simulink model "Closed Loop Control of Separately Excited DC Motor_Block_diagram"  (R2023b)
settings: Solver=VariableStepAuto  StartTime=0.0  StopTime=2  MaxStep=1e-6  RelTol=1e-6
libraries: simulink x1, slpidlib x1
settings Model: SimulationMode=accelerator  Creator=pradnya  LastModifiedBy=Asus
settings SolverCC: AlgebraicLoopSolver=TrustRegion
settings DataIOCC: ReturnWorkspaceOutputs=off
settings DebuggingCC: UnconnectedInputMsg=warning  UnconnectedOutputMsg=warning  UnconnectedLineMsg=warning  ArithmeticOperatorsInVariantConditions=warning
settings ModelReferenceCC: EnableRefExpFcnMdlSchedulingChecks=on
settings SFSimCC: SimUseLocalCustomCode=off  CustomCodeUndefinedFunction=UseInterfaceOnly
settings RTWCC: RTWUseLocalCustomCode=off

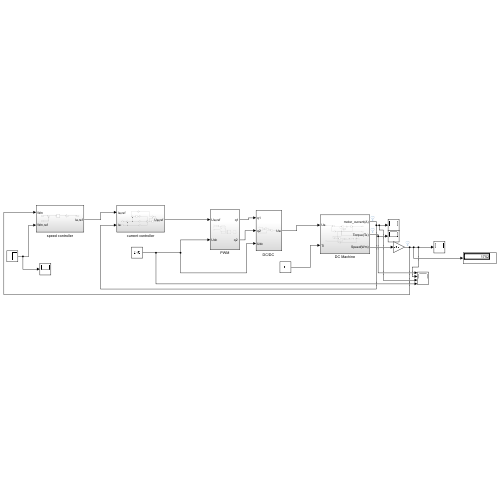
[thumbnail: Simulink's stored preview of the top-level diagram]
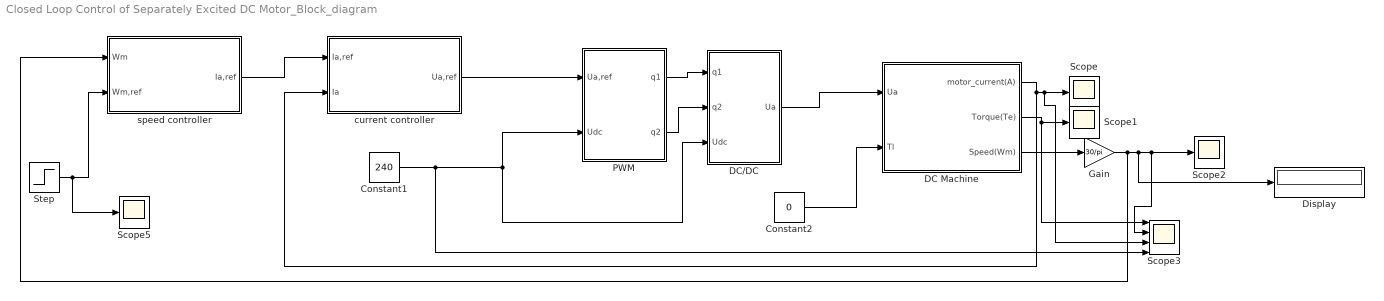
== system Closed Loop Control of Separately Excited DC Motor_Block_diagram ==
  Constant1 : Constant  Value=240
  Constant2 : Constant  Value=0
  "DC Machine " : Subsystem
  "DC/DC " : Subsystem
  Display : Display
  Gain : Gain  Gain=30/pi
  PWM : Subsystem
  Scope{,1..2,5} (4 alike) : Scope
  Scope3 : Scope  NumInputPorts=4
  Step : Step  Time=0.25  Before=875  After=1750  SampleTime=0.5
  current controller : Subsystem
  "speed controller " : Subsystem
  wires:
  "DC Machine "/3(Speed(Wm)) -> Gain/1
  "DC Machine "/2(Torque(Te)) -> Scope3/1, Scope1/1
  "DC Machine "/1(motor_current(A)) -> current controller/2(Ia), Scope3/3, Scope/1
  Gain/1 -> "speed controller "/1(Wm), Display/1, Scope3/2, Scope2/1
  PWM/1(q1) -> "DC/DC "/1(q1)
  PWM/2("q2 ") -> "DC/DC "/2(q2)
  Constant1/1 -> Scope3/4, PWM/2(Udc), "DC/DC "/3(Udc)
  Constant2/1 -> "DC Machine "/2(Tl)
  Step/1 -> Scope5/1, "speed controller "/2("Wm,ref ")
  current controller/1(Ua,ref) -> PWM/1(Ua,ref)
  "DC/DC "/1(Ua) -> "DC Machine "/1("Ua ")
  "speed controller "/1(Ia,ref) -> current controller/1("Ia,ref ")

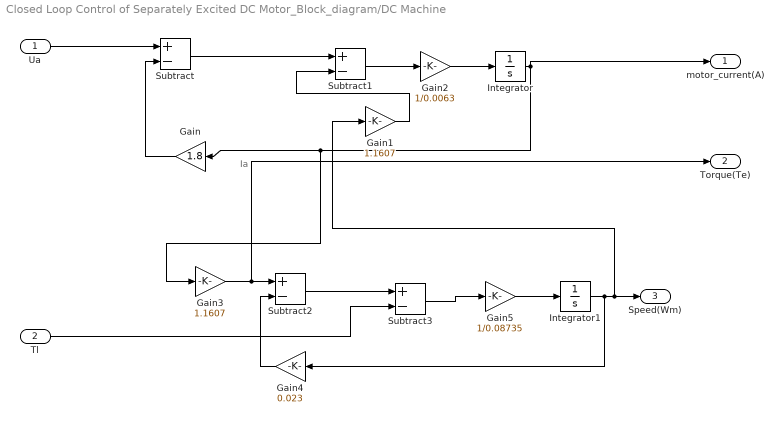
== system Closed Loop Control of Separately Excited DC Motor_Block_diagram/DC Machine  ==
  note: Ia
  "Ua " : Inport
  Tl : Inport  Port=2
  Gain : Gain  Gain=1.8
  Gain1 : Gain  Gain=1.1607
  Gain2 : Gain  Gain=1/0.0063
  Gain3 : Gain  Gain=1.1607
  Gain4 : Gain  Gain=0.023
  Gain5 : Gain  Gain=1/0.08735
  Integrator : Integrator
  Integrator1 : Integrator
  Subtract{,1..3} (4 alike) : Sum  Inputs=+-
  motor_current(A) : Outport  VectorParamsAs1DForOutWhenUnconnected=off
  Torque(Te) : Outport  Port=2  VectorParamsAs1DForOutWhenUnconnected=off
  Speed(Wm) : Outport  Port=3  VectorParamsAs1DForOutWhenUnconnected=off
  wires:
  Subtract1/1 -> Gain2/1
  Gain3/1 -> Torque(Te)/1, Subtract2/1
  Integrator/1 -> motor_current(A)/1, Gain3/1, Gain/1
  Gain2/1 -> Integrator/1
  Gain5/1 -> Integrator1/1
  Subtract/1 -> Subtract1/1
  Integrator1/1 -> Speed(Wm)/1, Gain1/1, Gain4/1
  Gain/1 -> Subtract/2
  Gain4/1 -> Subtract2/2
  Subtract2/1 -> Subtract3/1
  Subtract3/1 -> Gain5/1
  Gain1/1 -> Subtract1/2
  Tl/1 -> Subtract3/2
  "Ua "/1 -> Subtract/1

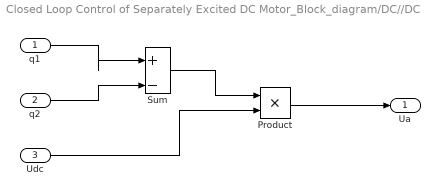
== system Closed Loop Control of Separately Excited DC Motor_Block_diagram/DC//DC  ==
  q1 : Inport
  q2 : Inport  Port=2
  Udc : Inport  Port=3
  Product : Product
  Sum : Sum  Inputs=|+-
  Ua : Outport  VectorParamsAs1DForOutWhenUnconnected=off
  wires:
  q1/1 -> Sum/1
  q2/1 -> Sum/2
  Sum/1 -> Product/1
  Udc/1 -> Product/2
  Product/1 -> Ua/1

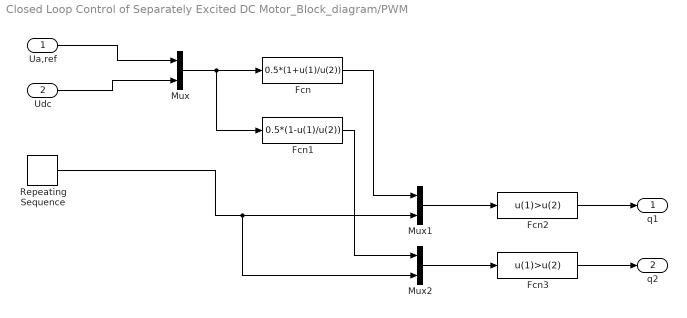
== system Closed Loop Control of Separately Excited DC Motor_Block_diagram/PWM ==
  Ua,ref : Inport
  Udc : Inport  Port=2
  Fcn : Fcn  Expr=0.5*(1+u(1)/u(2))
  Fcn1 : Fcn  Expr=0.5*(1-u(1)/u(2))
  Fcn2 : Fcn  Expr=u(1)>u(2)
  Fcn3 : Fcn  Expr=u(1)>u(2)
  Mux : Mux  Inputs=2
  Mux1 : Mux  Inputs=2
  Mux2 : Mux  Inputs=2
  Repeating Sequence : simulink/Sources/Repeating Sequence  rep_seq_t=[0 100e-6 200e-6]  rep_seq_y=[1 0 1]
  q1 : Outport  VectorParamsAs1DForOutWhenUnconnected=off
  "q2 " : Outport  Port=2  VectorParamsAs1DForOutWhenUnconnected=off
  wires:
  Ua,ref/1 -> Mux/1
  Udc/1 -> Mux/2
  Mux/1 -> Fcn1/1, Fcn/1
  Fcn/1 -> Mux1/1
  Fcn1/1 -> Mux2/1
  Repeating Sequence/1 -> Mux2/2, Mux1/2
  Mux1/1 -> Fcn2/1
  Mux2/1 -> Fcn3/1
  Fcn2/1 -> q1/1
  Fcn3/1 -> "q2 "/1

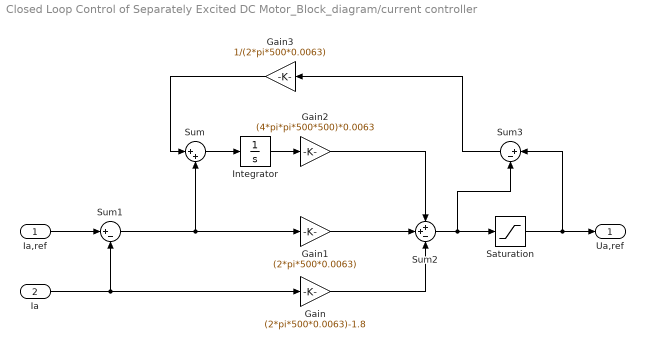
== system Closed Loop Control of Separately Excited DC Motor_Block_diagram/current controller ==
  "Ia,ref " : Inport
  Ia : Inport  Port=2
  Gain : Gain  Gain=(2*pi*500*0.0063)-1.8
  Gain1 : Gain  Gain=(2*pi*500*0.0063)
  Gain2 : Gain  Gain=(4*pi*pi*500*500)*0.0063
  Gain3 : Gain  Gain=1/(2*pi*500*0.0063)
  Integrator : Integrator
  Saturation : Saturate  UpperLimit=220  LowerLimit=-220
  Sum : Sum  Inputs=|++
  Sum1 : Sum  Inputs=|+-
  Sum2 : Sum  Inputs=++-
  Sum3 : Sum  Inputs=|+-
  Ua,ref : Outport  VectorParamsAs1DForOutWhenUnconnected=off
  wires:
  "Ia,ref "/1 -> Sum1/1
  Ia/1 -> Gain/1, Sum1/2
  Sum1/1 -> Sum/2, Gain1/1
  Gain3/1 -> Sum/1
  Sum/1 -> Integrator/1
  Integrator/1 -> Gain2/1
  Gain1/1 -> Sum2/2
  Gain2/1 -> Sum2/1
  Gain/1 -> Sum2/3
  Sum2/1 -> Sum3/2, Saturation/1
  Saturation/1 -> Sum3/1, Ua,ref/1
  Sum3/1 -> Gain3/1

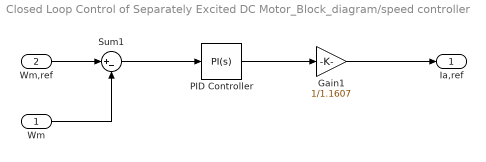
== system Closed Loop Control of Separately Excited DC Motor_Block_diagram/speed controller  ==
  Wm : Inport
  "Wm,ref " : Inport  Port=2
  Gain1 : Gain  Gain=1/1.1607
  PID Controller : slpidlib/PID Controller  Controller=PI  Form=Parallel  TimeDomain=Continuous-time  UseExternalTs=off  SampleTime=-1  IntegratorMethod=Forward Euler  FilterMethod=Forward Euler  ControllerParametersSource=internal  P=5  I=0.1  UseKiTs=off  D=0  N=100  UseFilter=on  TunerSelectOption=Transfer Function Based (PID Tuner App)  InitialConditionSource=internal  InitialConditionForIntegrator=0  InitialConditionForFilter=0  DifferentiatorICPrevScaledInput=0  ExternalReset=none  TrackingMode=off  Kt=1  LimitOutput=off  SatLimitsSource=internal  UpperSaturationLimit=inf  LowerSaturationLimit=-inf  LinearizeAsGain=on  AntiWindupMode=none  Kb=1  LimitIntegrator=off  UpperIntegratorSaturationLimit=inf  LowerIntegratorSaturationLimit=-inf  POutMin=[]  POutMax=[]  IOutMin=[]  IOutMax=[]  DOutMin=[]  DOutMax=[]  NOutMin=[]  NOutMax=[]  SumOutMin=[]  SumOutMax=[]  SaturationOutMin=[]  SaturationOutMax=[]  PParamMin=[]  PParamMax=[]  IParamMin=[]  IParamMax=[]  DParamMin=[]  DParamMax=[]  NParamMin=[]  NParamMax=[]  KbParamMin=[]  KbParamMax=[]  KtParamMin=[]  KtParamMax=[]  KbOutMin=[]  KbOutMax=[]  KtOutMin=[]  KtOutMax=[]  IntegratorOutMin=[]  IntegratorOutMax=[]  FilterOutMin=[]  FilterOutMax=[]  SumI1OutMin=[]  SumI1OutMax=[]  SumI2OutMin=[]  SumI2OutMax=[]  SumI3OutMin=[]  SumI3OutMax=[]  SumI4OutMin=[]  SumI4OutMax=[]  SumDOutMin=[]  SumDOutMax=[]  DifferentiatorOutMin=[]  DifferentiatorOutMax=[]  FilterDiffOutCoefMin=[]  FilterDiffOutCoefMax=[]  ReciprocalOutMin=[]  ReciprocalOutMax=[]  SumDenOutMin=[]  SumDenOutMax=[]  SumNumOutMin=[]  SumNumOutMax=[]  DivideOutMin=[]  DivideOutMax=[]  UdiffTsProdOutMin=[]  UdiffTsProdOutMax=[]  NTsProdOutMin=[]  NTsProdOutMax=[]  UintegralTsProdOutMin=[]  UintegralTsProdOutMax=[]  UngainTsProdOutMin=[]  UngainTsProdOutMax=[]  ClampingZeroOutDataTypeStr=Inherit: Inherit via back propagation  ClampingZeroOutMin=[]  ClampingZeroOutMax=[]  FilterDenConstantOutDataTypeStr=Inherit: Inherit via back propagation  FilterDenConstantOutMin=[]  FilterDenConstantOutMax=[]  PCopyOutDataTypeStr=Inherit: Inherit via back propagation  PCopyOutMin=[]  PCopyOutMax=[]  NCopyOutDataTypeStr=Inherit: Inherit via back propagation  NCopyOutMin=[]  NCopyOutMax=[]  IntegratorContinuousStateAttributes=''  IntegratorStateMustResolveToSignalObject=off  IntegratorRTWStateStorageClass=Auto  FilterContinuousStateAttributes=''  FilterStateMustResolveToSignalObject=off  FilterRTWStateStorageClass=Auto  ParallelPVariant=InternalParameters  IdealPVariant=Disabled  IVariant=InternalParameters  DVariant=Disabled  IntegratorVariant=Continuous  SatVariant=Disabled  AWVariant=Passthrough  PCopyVariant=Disabled  TRVariant=Disabled  FdbkBlocksVariant=Forward  IdealPFdbkVariant=Disabled  SatFdbkVariant=Disabled  DerivativeFilterVariant=Disabled  NVariant=Disabled  NCopyVariant=Disabled_SignalSpec  FilterICVariant=Disabled  IntegratorICVariant=InternalICs  ExternalResetVariant=Disabled  TRSumVariant=Passthrough  SumFdbkVariant=Disabled  SumVariant=Sum_PI  TsampFilterVariant=InternalTs  TsampNgainVariant=Passthrough  TsampIntegralVariant=Disabled_SignalSpec  ExternalSaturationOutDataTypeStr=Inherit: Same as second input
  Sum1 : Sum  Inputs=|+-
  Ia,ref : Outport  VectorParamsAs1DForOutWhenUnconnected=off
  wires:
  "Wm,ref "/1 -> Sum1/1
  Wm/1 -> Sum1/2
  Sum1/1 -> PID Controller/1
  PID Controller/1 -> Gain1/1
  Gain1/1 -> Ia,ref/1
